simulink model "Plant_Model_Gathering"  (R2023a)
settings: Solver=VariableStepAuto  StartTime=0.0  StopTime=10.0  RelTol=1e-3
undefined symbols (not defined in the file): Amps, Ax, Ay, b, d, g, Ion, Ixx, Izz, Jr, Lithium, m, PD
libraries: simulink x5, spsBatteryLib x1, spsControlledCurrentSourceLib x1, spsCurrentMeasurementLib x1
settings Model: Creator=NADJICH  LastModifiedBy=NADJICH

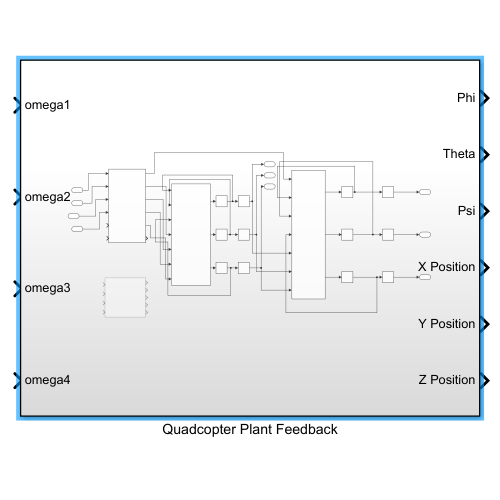
[thumbnail: Simulink's stored preview of the top-level diagram]
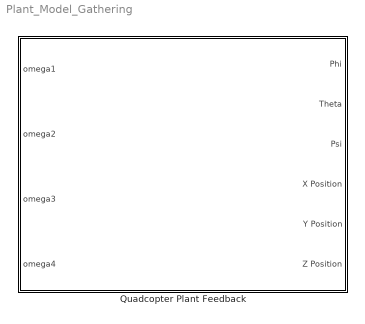
== system Plant_Model_Gathering ==
  Quadcopter Plant Feedback : Subsystem

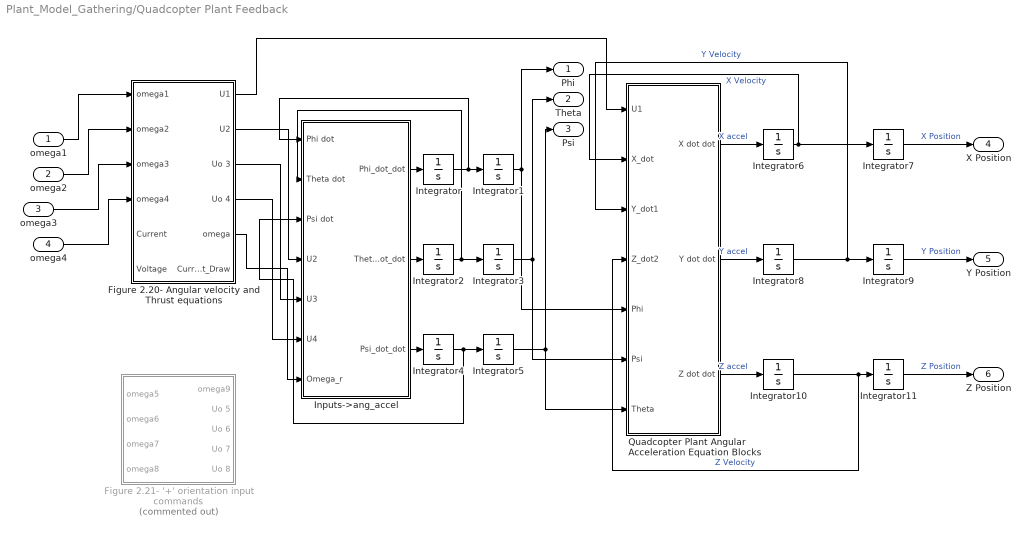
== system Plant_Model_Gathering/Quadcopter Plant Feedback ==
  omega1 : Inport
  omega2 : Inport  Port=2
  omega3 : Inport  Port=3
  omega4 : Inport  Port=4
  Figure 2.20- Angular velocity and Thrust equations : Subsystem
  Figure 2.21- '+' orientation input commands : Subsystem  Commented=on
  Inputs->ang_accel : Subsystem
  Integrator{,2,4,6..10} (8 alike) : Integrator
  Integrator1 : Integrator  WrapState=on
  Integrator11 : Integrator  LimitOutput=on  UpperSaturationLimit=0
  Integrator3 : Integrator  WrapState=on
  Integrator5 : Integrator  WrapState=on
  Quadcopter Plant Angular Acceleration Equation Blocks : Subsystem
  Phi : Outport
  Theta : Outport  Port=2
  Psi : Outport  Port=3
  X Position : Outport  Port=4
  Y Position : Outport  Port=5
  Z Position : Outport  Port=6
  wires:
  omega1/1 -> Figure 2.20- Angular velocity and Thrust equations/1(omega1)
  omega2/1 -> Figure 2.20- Angular velocity and Thrust equations/2(omega2)
  omega3/1 -> Figure 2.20- Angular velocity and Thrust equations/3(omega3)
  omega4/1 -> Figure 2.20- Angular velocity and Thrust equations/4(omega4)
  Figure 2.20- Angular velocity and Thrust equations/5(omega) -> Inputs->ang_accel/7(Omega_r)
  Figure 2.20- Angular velocity and Thrust equations/2(U2) -> Inputs->ang_accel/4(U2)
  Figure 2.20- Angular velocity and Thrust equations/3(Uo 3) -> Inputs->ang_accel/5(U3)
  Figure 2.20- Angular velocity and Thrust equations/4(Uo 4) -> Inputs->ang_accel/6(U4)
  Inputs->ang_accel/1(Phi_dot_dot) -> Integrator/1
  Integrator/1 -> Integrator1/1, Inputs->ang_accel/1(Phi dot)
  Integrator2/1 -> Integrator3/1, Inputs->ang_accel/2(Theta dot)
  Integrator4/1 -> Integrator5/1, Inputs->ang_accel/3(Psi dot)
  Inputs->ang_accel/2(Theta_dot_dot) -> Integrator2/1
  Inputs->ang_accel/3(Psi_dot_dot) -> Integrator4/1
  Integrator1/1 -> Phi/1, Quadcopter Plant Angular Acceleration Equation Blocks/5(Phi)
  Integrator3/1 -> Theta/1, Quadcopter Plant Angular Acceleration Equation Blocks/6(Psi)
  Integrator5/1 -> Psi/1, Quadcopter Plant Angular Acceleration Equation Blocks/7(Theta)
  Figure 2.20- Angular velocity and Thrust equations/1(U1) -> Quadcopter Plant Angular Acceleration Equation Blocks/1(U1)
  Quadcopter Plant Angular Acceleration Equation Blocks/1(X dot dot) -> Integrator6/1  "X accel"
  Quadcopter Plant Angular Acceleration Equation Blocks/2(Y dot dot) -> Integrator8/1  "Y accel"
  Quadcopter Plant Angular Acceleration Equation Blocks/3(Z dot dot) -> Integrator10/1  "Z accel"
  Integrator6/1 -> Quadcopter Plant Angular Acceleration Equation Blocks/2(X_dot), Integrator7/1  "X Velocity"
  Integrator7/1 -> X Position/1  "X Position"
  Integrator8/1 -> Quadcopter Plant Angular Acceleration Equation Blocks/3(Y_dot1), Integrator9/1  "Y Velocity"
  Integrator9/1 -> Y Position/1  "Y Position"
  Integrator10/1 -> Integrator11/1, Quadcopter Plant Angular Acceleration Equation Blocks/4(Z_dot2)  "Z Velocity"
  Integrator11/1 -> Z Position/1  "Z Position"

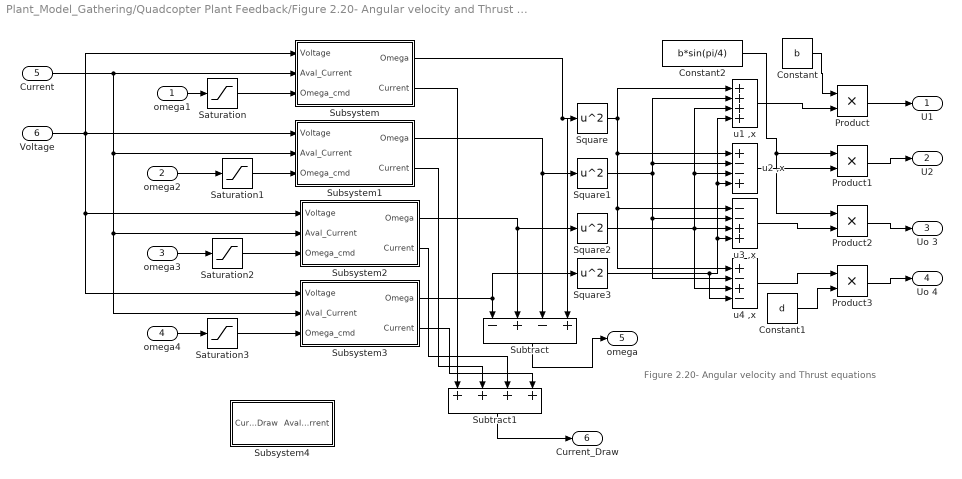
== system Plant_Model_Gathering/Quadcopter Plant Feedback/Figure 2.20- Angular velocity and Thrust equations ==
  note: Figure 2.20- Angular velocity and Thrust equations
  omega1 : Inport
  omega2 : Inport  Port=2
  omega3 : Inport  Port=3
  omega4 : Inport  Port=4
  Current : Inport  Port=5
  Voltage : Inport  Port=6
  Constant : Constant  Value=b
  Constant1 : Constant  Value=d
  Constant2 : Constant  Value=b*sin(pi/4)
  Product{,1..3} (4 alike) : Product
  Saturation{,1..3} (4 alike) : Saturate  UpperLimit=inf  LowerLimit=0
  Square{,1..3} (4 alike) : Math  Operator=square
  Subsystem : Subsystem  mask{Jr=6.5e-7, b_m=2.415-6, Kemf=0.00255, Kt=0.00255, R=0.117, L=1.17e-4}
  Subsystem1 : Subsystem  mask{Jr=6.5e-7, b_m=2.415-6, Kemf=0.00255, Kt=0.00255, R=0.117, L=1.17e-4}
  Subsystem2 : Subsystem  mask{Jr=6.5e-7, b_m=2.415-6, Kemf=0.00255, Kt=0.00255, R=0.117, L=1.17e-4}
  Subsystem3 : Subsystem  mask{Jr=6.5e-7, b_m=2.415-6, Kemf=0.00255, Kt=0.00255, R=0.117, L=1.17e-4}
  Subsystem4 : Subsystem
  Subtract : Sum  Inputs=-+-+
  Subtract1 : Sum  Inputs=++++
  u1 ,x : Sum  Inputs=++++
  u2 ,x : Sum  Inputs=+--+
  u3 ,x : Sum  Inputs=--++
  u4 ,x : Sum  Inputs=+-+-
  U1 : Outport
  U2 : Outport  Port=2
  Uo 3 : Outport  Port=3
  Uo 4 : Outport  Port=4
  omega : Outport  Port=5
  Current_Draw : Outport  Port=6
  wires:
  Constant/1 -> Product/1
  Product1/1 -> U2/1
  u4 ,x/1 -> Product3/1
  Square3/1 -> u4 ,x/4, u3 ,x/4, u2 ,x/4, u1 ,x/4
  omega1/1 -> Saturation/1
  Product/1 -> U1/1
  Square1/1 -> u2 ,x/2, u1 ,x/2, u4 ,x/2, u3 ,x/2
  u3 ,x/1 -> Product2/2
  u1 ,x/1 -> Product/2
  Constant1/1 -> Product3/2
  Constant2/1 -> Product1/1, Product2/1
  Square/1 -> u4 ,x/1, u3 ,x/1, u2 ,x/1, u1 ,x/1
  Square2/1 -> u4 ,x/3, u3 ,x/3, u1 ,x/3, u2 ,x/3
  Product2/1 -> Uo 3/1
  Subtract/1 -> omega/1
  Product3/1 -> Uo 4/1
  u2 ,x/1 -> Product1/2
  omega2/1 -> Saturation1/1
  omega3/1 -> Saturation2/1
  omega4/1 -> Saturation3/1
  Subsystem/1(Omega) -> Square/1, Subtract/4
  Subsystem1/1(Omega) -> Subtract/3, Square1/1
  Subsystem2/1(Omega) -> Subtract/2, Square2/1
  Subsystem3/1(Omega) -> Square3/1, Subtract/1
  Subsystem/2(Current) -> Subtract1/1
  Subsystem1/2(Current) -> Subtract1/2
  Subsystem2/2(Current) -> Subtract1/3
  Subsystem3/2(Current) -> Subtract1/4
  Subtract1/1 -> Current_Draw/1
  Current/1 -> Subsystem/2(Aval_Current), Subsystem1/2(Aval_Current), Subsystem2/2(Aval_Current), Subsystem3/2(Aval_Current)
  Voltage/1 -> Subsystem/1(Voltage), Subsystem1/1(Voltage), Subsystem2/1(Voltage), Subsystem3/1(Voltage)
  Saturation/1 -> Subsystem/3(Omega_cmd)
  Saturation1/1 -> Subsystem1/3(Omega_cmd)
  Saturation2/1 -> Subsystem2/3(Omega_cmd)
  Saturation3/1 -> Subsystem3/3(Omega_cmd)

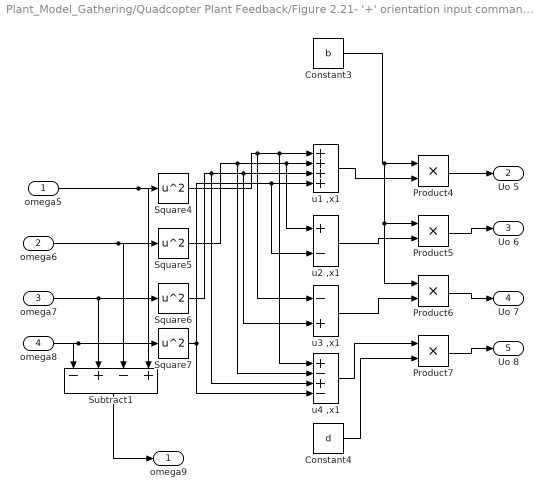
== system Plant_Model_Gathering/Quadcopter Plant Feedback/Figure 2.21- '+' orientation input commands ==
  omega5 : Inport
  omega6 : Inport  Port=2
  omega7 : Inport  Port=3
  omega8 : Inport  Port=4
  Constant3 : Constant  Value=b
  Constant4 : Constant  Value=d
  Product{4..7} (4 alike) : Product
  Square{4..7} (4 alike) : Math  Operator=square
  Subtract1 : Sum  Inputs=-+-+
  u1 ,x1 : Sum  Inputs=++++
  u2 ,x1 : Sum  Inputs=+-
  u3 ,x1 : Sum  Inputs=-+
  u4 ,x1 : Sum  Inputs=+-+-
  omega9 : Outport
  Uo 5 : Outport  Port=2
  Uo 6 : Outport  Port=3
  Uo 7 : Outport  Port=4
  Uo 8 : Outport  Port=5
  wires:
  Square5/1 -> u4 ,x1/2, u2 ,x1/1, u1 ,x1/2
  Constant3/1 -> Product6/1, Product5/1, Product4/1
  Square4/1 -> u3 ,x1/1, u4 ,x1/1, u1 ,x1/1
  Product7/1 -> Uo 8/1
  Constant4/1 -> Product7/2
  omega6/1 -> Square5/1, Subtract1/3
  Product5/1 -> Uo 6/1
  Square7/1 -> u2 ,x1/2, u1 ,x1/4, u4 ,x1/4
  Product4/1 -> Uo 5/1
  u1 ,x1/1 -> Product4/2
  Square6/1 -> u4 ,x1/3, u3 ,x1/2, u1 ,x1/3
  omega8/1 -> Square7/1, Subtract1/1
  u2 ,x1/1 -> Product5/2
  Subtract1/1 -> omega9/1
  omega7/1 -> Square6/1, Subtract1/2
  omega5/1 -> Subtract1/4, Square4/1
  u3 ,x1/1 -> Product6/2
  Product6/1 -> Uo 7/1
  u4 ,x1/1 -> Product7/1

== system Plant_Model_Gathering/Quadcopter Plant Feedback/Inputs->ang_accel ==
  Phi dot : Inport
  Theta dot : Inport  Port=2
  Psi dot : Inport  Port=3
  U2 : Inport  Port=4
  U3 : Inport  Port=5
  U4 : Inport  Port=6
  Omega_r : Inport  Port=7
  Subsystem2 : Subsystem
  Subsystem3 : Subsystem
  Subsystem4 : Subsystem
  Phi_dot_dot : Outport
  Theta_dot_dot : Outport  Port=2
  Psi_dot_dot : Outport  Port=3
  wires:
  Subsystem4/1(Psi_dot_dot) -> Psi_dot_dot/1
  Psi dot/1 -> Subsystem3/4(Omega_r), Subsystem2/4(Psi dot)
  Phi dot/1 -> Subsystem3/2(Phi dot), Subsystem4/3(Phi dot)
  Omega_r/1 -> Subsystem3/1(Psi dot), Subsystem2/2(omega)
  Subsystem3/1(Theta_dot_dot) -> Theta_dot_dot/1
  Subsystem2/1(Phi_dot_dot) -> Phi_dot_dot/1
  Theta dot/1 -> Subsystem2/3(Theta dot), Subsystem4/2(Theta dot)
  U4/1 -> Subsystem4/1(In1)
  U2/1 -> Subsystem2/1(U2)
  U3/1 -> Subsystem3/3(U3)

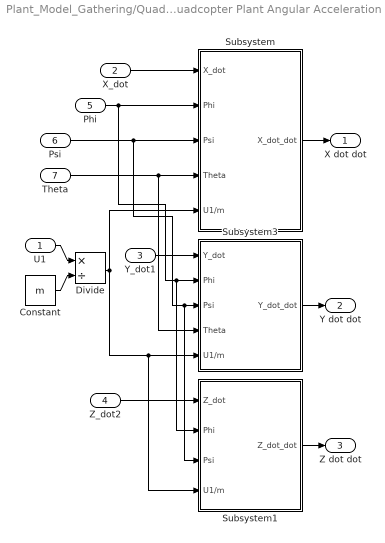
== system Plant_Model_Gathering/Quadcopter Plant Feedback/Quadcopter Plant Angular Acceleration Equation Blocks ==
  U1 : Inport
  X_dot : Inport  Port=2
  Y_dot1 : Inport  Port=3
  Z_dot2 : Inport  Port=4
  Phi : Inport  Port=5
  Psi : Inport  Port=6
  Theta : Inport  Port=7
  Constant : Constant  Value=m
  Divide : Product  Inputs=*/
  Subsystem : Subsystem
  Subsystem1 : Subsystem
  Subsystem3 : Subsystem
  X dot dot : Outport
  Y dot dot : Outport  Port=2
  Z dot dot : Outport  Port=3
  wires:
  Subsystem3/1(Y_dot_dot) -> Y dot dot/1
  U1/1 -> Divide/1
  Constant/1 -> Divide/2
  Subsystem/1(X_dot_dot) -> X dot dot/1
  Subsystem1/1(Z_dot_dot) -> Z dot dot/1
  X_dot/1 -> Subsystem/1(X_dot)
  Divide/1 -> Subsystem1/4(U1/m), Subsystem3/5(U1/m), Subsystem/5(U1/m)
  Y_dot1/1 -> Subsystem3/1(Y_dot)
  Phi/1 -> Subsystem1/2(Phi), Subsystem3/2(Phi), Subsystem/2(Phi)
  Theta/1 -> Subsystem3/4(Theta), Subsystem/4(Theta)
  Psi/1 -> Subsystem1/3(Psi), Subsystem3/3(Psi), Subsystem/3(Psi)
  Z_dot2/1 -> Subsystem1/1(Z_dot)

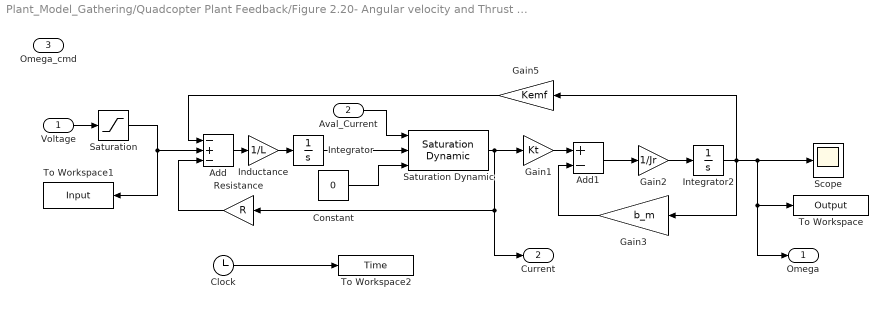
== system Plant_Model_Gathering/Quadcopter Plant Feedback/Figure 2.20- Angular velocity and Thrust equations/Subsystem ==
  Voltage : Inport
  Aval_Current : Inport  Port=2
  Omega_cmd : Inport  Port=3
  Add : Sum  Inputs=-+-
  Add1 : Sum  Inputs=+-
  Clock : Clock
  Constant : Constant  Value=0
  Gain1 : Gain  Gain=Kt
  Gain2 : Gain  Gain=1/Jr
  Gain3 : Gain  Gain=b_m
  Gain5 : Gain  Gain=Kemf
  Inductance : Gain  Gain=1/L
  Integrator : Integrator  LimitOutput=on  UpperSaturationLimit=0
  Integrator2 : Integrator  LimitOutput=on  UpperSaturationLimit=0
  Resistance : Gain  Gain=R
  Saturation : Saturate
  Saturation Dynamic : simulink/Discontinuities/Saturation Dynamic  OutMin=[]  OutMax=[]  OutDataTypeStr=Inherit: Same as second input  OutDataType=fixdt(1, 16)  OutScaling=2^-10  DoSatur=off
  Scope : Scope
  To Workspace : ToWorkspace  VariableName=Output  SampleTime=-1
  To Workspace1 : ToWorkspace  VariableName=Input  SampleTime=-1
  To Workspace2 : ToWorkspace  VariableName=Time  SampleTime=-1
  Omega : Outport
  Current : Outport  Port=2
  wires:
  Voltage/1 -> Saturation/1
  Integrator/1 -> Saturation Dynamic/2
  Integrator2/1 -> Scope/1, Omega/1, To Workspace/1, Gain3/1, Gain5/1
  Add/1 -> Inductance/1
  Gain2/1 -> Integrator2/1
  Gain5/1 -> Add/1
  Gain3/1 -> Add1/2
  Add1/1 -> Gain2/1
  Resistance/1 -> Add/3
  Inductance/1 -> Integrator/1
  Gain1/1 -> Add1/1
  Saturation/1 -> Add/2, To Workspace1/1
  Clock/1 -> To Workspace2/1
  Saturation Dynamic/1 -> Current/1, Resistance/1, Gain1/1
  Constant/1 -> Saturation Dynamic/3
  Aval_Current/1 -> Saturation Dynamic/1

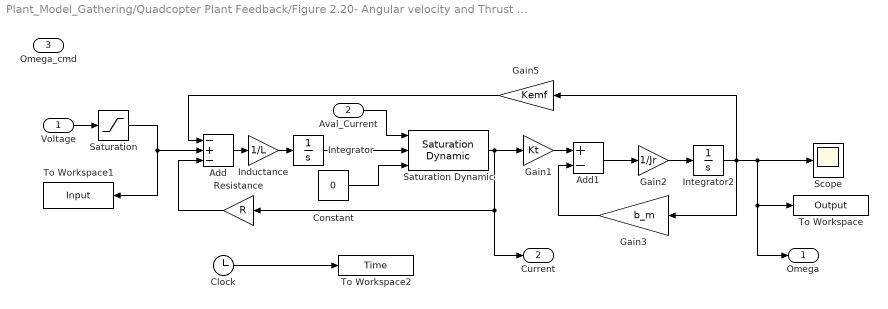
== system Plant_Model_Gathering/Quadcopter Plant Feedback/Figure 2.20- Angular velocity and Thrust equations/Subsystem1 ==
  Voltage : Inport
  Aval_Current : Inport  Port=2
  Omega_cmd : Inport  Port=3
  Add : Sum  Inputs=-+-
  Add1 : Sum  Inputs=+-
  Clock : Clock
  Constant : Constant  Value=0
  Gain1 : Gain  Gain=Kt
  Gain2 : Gain  Gain=1/Jr
  Gain3 : Gain  Gain=b_m
  Gain5 : Gain  Gain=Kemf
  Inductance : Gain  Gain=1/L
  Integrator : Integrator  LimitOutput=on  UpperSaturationLimit=0
  Integrator2 : Integrator  LimitOutput=on  UpperSaturationLimit=0
  Resistance : Gain  Gain=R
  Saturation : Saturate
  Saturation Dynamic : simulink/Discontinuities/Saturation Dynamic  OutMin=[]  OutMax=[]  OutDataTypeStr=Inherit: Same as second input  OutDataType=fixdt(1, 16)  OutScaling=2^-10  DoSatur=off
  Scope : Scope
  To Workspace : ToWorkspace  VariableName=Output  SampleTime=-1
  To Workspace1 : ToWorkspace  VariableName=Input  SampleTime=-1
  To Workspace2 : ToWorkspace  VariableName=Time  SampleTime=-1
  Omega : Outport
  Current : Outport  Port=2
  wires:
  Aval_Current/1 -> Saturation Dynamic/1
  Constant/1 -> Saturation Dynamic/3
  Saturation Dynamic/1 -> Gain1/1, Resistance/1, Current/1
  Clock/1 -> To Workspace2/1
  Saturation/1 -> To Workspace1/1, Add/2
  Gain1/1 -> Add1/1
  Inductance/1 -> Integrator/1
  Resistance/1 -> Add/3
  Add1/1 -> Gain2/1
  Gain3/1 -> Add1/2
  Gain5/1 -> Add/1
  Gain2/1 -> Integrator2/1
  Add/1 -> Inductance/1
  Integrator2/1 -> Gain5/1, Gain3/1, To Workspace/1, Omega/1, Scope/1
  Integrator/1 -> Saturation Dynamic/2
  Voltage/1 -> Saturation/1

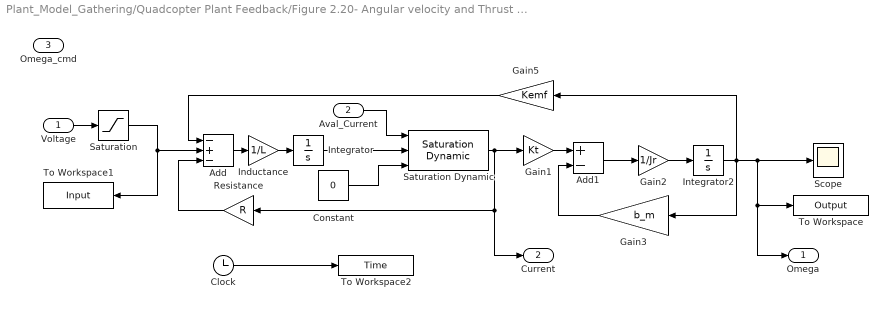
== system Plant_Model_Gathering/Quadcopter Plant Feedback/Figure 2.20- Angular velocity and Thrust equations/Subsystem2 ==
  Voltage : Inport
  Aval_Current : Inport  Port=2
  Omega_cmd : Inport  Port=3
  Add : Sum  Inputs=-+-
  Add1 : Sum  Inputs=+-
  Clock : Clock
  Constant : Constant  Value=0
  Gain1 : Gain  Gain=Kt
  Gain2 : Gain  Gain=1/Jr
  Gain3 : Gain  Gain=b_m
  Gain5 : Gain  Gain=Kemf
  Inductance : Gain  Gain=1/L
  Integrator : Integrator  LimitOutput=on  UpperSaturationLimit=0
  Integrator2 : Integrator  LimitOutput=on  UpperSaturationLimit=0
  Resistance : Gain  Gain=R
  Saturation : Saturate
  Saturation Dynamic : simulink/Discontinuities/Saturation Dynamic  OutMin=[]  OutMax=[]  OutDataTypeStr=Inherit: Same as second input  OutDataType=fixdt(1, 16)  OutScaling=2^-10  DoSatur=off
  Scope : Scope
  To Workspace : ToWorkspace  VariableName=Output  SampleTime=-1
  To Workspace1 : ToWorkspace  VariableName=Input  SampleTime=-1
  To Workspace2 : ToWorkspace  VariableName=Time  SampleTime=-1
  Omega : Outport
  Current : Outport  Port=2
  wires:
  Voltage/1 -> Saturation/1
  Integrator/1 -> Saturation Dynamic/2
  Integrator2/1 -> Scope/1, Omega/1, To Workspace/1, Gain3/1, Gain5/1
  Add/1 -> Inductance/1
  Gain2/1 -> Integrator2/1
  Gain5/1 -> Add/1
  Gain3/1 -> Add1/2
  Add1/1 -> Gain2/1
  Resistance/1 -> Add/3
  Inductance/1 -> Integrator/1
  Gain1/1 -> Add1/1
  Saturation/1 -> Add/2, To Workspace1/1
  Clock/1 -> To Workspace2/1
  Saturation Dynamic/1 -> Current/1, Resistance/1, Gain1/1
  Constant/1 -> Saturation Dynamic/3
  Aval_Current/1 -> Saturation Dynamic/1

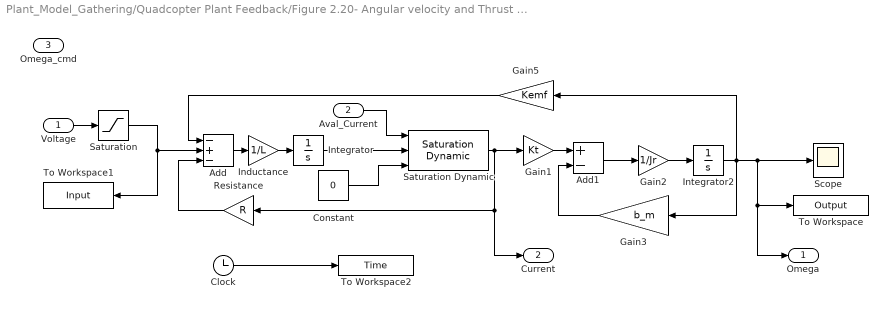
== system Plant_Model_Gathering/Quadcopter Plant Feedback/Figure 2.20- Angular velocity and Thrust equations/Subsystem3 ==
  Voltage : Inport
  Aval_Current : Inport  Port=2
  Omega_cmd : Inport  Port=3
  Add : Sum  Inputs=-+-
  Add1 : Sum  Inputs=+-
  Clock : Clock
  Constant : Constant  Value=0
  Gain1 : Gain  Gain=Kt
  Gain2 : Gain  Gain=1/Jr
  Gain3 : Gain  Gain=b_m
  Gain5 : Gain  Gain=Kemf
  Inductance : Gain  Gain=1/L
  Integrator : Integrator  LimitOutput=on  UpperSaturationLimit=0
  Integrator2 : Integrator  LimitOutput=on  UpperSaturationLimit=0
  Resistance : Gain  Gain=R
  Saturation : Saturate
  Saturation Dynamic : simulink/Discontinuities/Saturation Dynamic  OutMin=[]  OutMax=[]  OutDataTypeStr=Inherit: Same as second input  OutDataType=fixdt(1, 16)  OutScaling=2^-10  DoSatur=off
  Scope : Scope
  To Workspace : ToWorkspace  VariableName=Output  SampleTime=-1
  To Workspace1 : ToWorkspace  VariableName=Input  SampleTime=-1
  To Workspace2 : ToWorkspace  VariableName=Time  SampleTime=-1
  Omega : Outport
  Current : Outport  Port=2
  wires:
  Aval_Current/1 -> Saturation Dynamic/1
  Constant/1 -> Saturation Dynamic/3
  Saturation Dynamic/1 -> Gain1/1, Resistance/1, Current/1
  Clock/1 -> To Workspace2/1
  Saturation/1 -> To Workspace1/1, Add/2
  Gain1/1 -> Add1/1
  Inductance/1 -> Integrator/1
  Resistance/1 -> Add/3
  Add1/1 -> Gain2/1
  Gain3/1 -> Add1/2
  Gain5/1 -> Add/1
  Gain2/1 -> Integrator2/1
  Add/1 -> Inductance/1
  Integrator2/1 -> Gain5/1, Gain3/1, To Workspace/1, Omega/1, Scope/1
  Integrator/1 -> Saturation Dynamic/2
  Voltage/1 -> Saturation/1

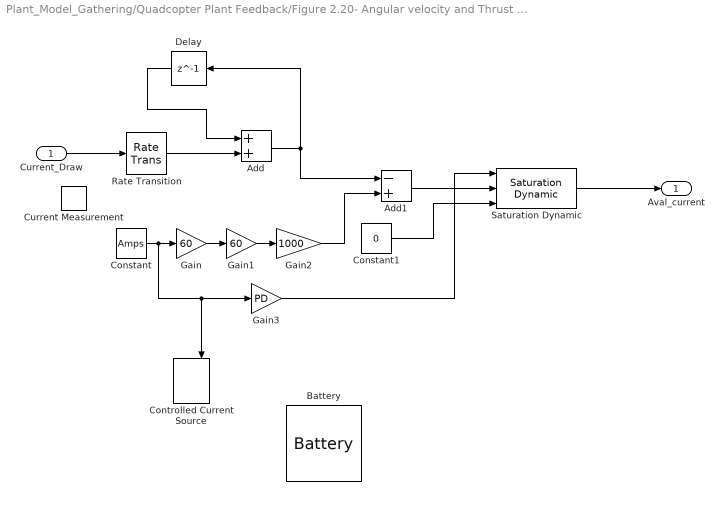
== system Plant_Model_Gathering/Quadcopter Plant Feedback/Figure 2.20- Angular velocity and Thrust equations/Subsystem4 ==
  Current_Draw : Inport
  Add : Sum
  Add1 : Sum  Inputs=-+
  Battery : spsBatteryLib/Battery  BatType=Lithium-Ion  ShowTempParam=off  ThermalPreset=no  ShowAgeParam=off  NomV=10  NomQ=0.7  SOC=100  Batt_Tr=30  PresetModel=on  MaxQ=0.7  MinV=7.5  FullV=11.6399  Dis_rate=0.30435  R=0.14286  Normal_OP=0.63304  expZone="[10.8039    0.0343913]"  current=[6.5 13 32.5]  Units=Time  Tci=20  NomT=20  T2=-30  MaxQ2=4.8  FullV2=7.1  Normal_OP2=5.655  expZone2="[6.58           1]"  Rca=0.6  ti=2000  Dp=0  Neq0=0  Tsim=1e6  Ta1=25  Qeol=5.4*0.9  Reol=0.013333*1.2  Char_age=[2.3478, 3]  Dis_age=[2.3478, 10]  N1=1500  N2=10500  N3=1000  N4=1400  Ta2=45  N5=950
  Constant : Constant  Value=Amps
  Constant1 : Constant  Value=0
  Controlled Current Source : spsControlledCurrentSourceLib/Controlled Current Source  Initialize=on  Source_Type=AC  Amplitude=0  Phase=0  Frequency=0  Measurements=None
  Current Measurement : spsCurrentMeasurementLib/Current Measurement  PhasorSimulation=off  OutputType=Complex  PSBequivalent=0
  Delay : Delay  DelayLength=1
  Gain : Gain  Gain=60
  Gain1 : Gain  Gain=60
  Gain2 : Gain  Gain=1000
  Gain3 : Gain  Gain=PD
  Rate Transition : RateTransition
  Saturation Dynamic : simulink/Discontinuities/Saturation Dynamic  OutMin=[]  OutMax=[]  OutDataTypeStr=Inherit: Same as second input  OutDataType=fixdt(1, 16)  OutScaling=2^-10  DoSatur=off
  Aval_current : Outport
  wires:
  Current_Draw/1 -> Rate Transition/1
  Add/1 -> Delay/1, Add1/1
  Delay/1 -> Add/1
  Rate Transition/1 -> Add/2
  Gain/1 -> Gain1/1
  Gain1/1 -> Gain2/1
  Constant/1 -> Controlled Current Source/1, Gain3/1, Gain/1
  Gain2/1 -> Add1/2
  Add1/1 -> Saturation Dynamic/2
  Gain3/1 -> Saturation Dynamic/1
  Constant1/1 -> Saturation Dynamic/3
  Saturation Dynamic/1 -> Aval_current/1

== system Plant_Model_Gathering/Quadcopter Plant Feedback/Inputs->ang_accel/Subsystem2 ==
  U2 : Inport
  omega : Inport  Port=2
  Theta dot : Inport  Port=3
  Psi dot : Inport  Port=4
  Add : Sum  Inputs=+++
  Constant : Constant
  Constant1 : Constant  Value=Jr
  Constant2 : Constant  Value=Izz-Ixx
  Constant3 : Constant
  Divide : Product  Inputs=*/
  Product : Product
  Product1 : Product  Inputs=3
  Product2 : Product  Inputs=3
  Phi_dot_dot : Outport
  wires:
  Add/1 -> Divide/1
  Divide/1 -> Phi_dot_dot/1
  Constant2/1 -> Product2/3
  Product2/1 -> Add/3
  U2/1 -> Product/2
  Product/1 -> Add/1
  Constant/1 -> Product/1
  Product1/1 -> Add/2
  Constant1/1 -> Product1/1
  Constant3/1 -> Divide/2
  omega/1 -> Product1/2
  Theta dot/1 -> Product2/1, Product1/3
  Psi dot/1 -> Product2/2

== system Plant_Model_Gathering/Quadcopter Plant Feedback/Inputs->ang_accel/Subsystem3 ==
  Psi dot : Inport
  Phi dot : Inport  Port=2
  U3 : Inport  Port=3
  Omega_r : Inport  Port=4
  Add2 : Sum  Inputs=+++
  Constant11 : Constant
  Constant12 : Constant  Value=Izz-Ixx
  Constant8 : Constant
  Constant9 : Constant  Value=Jr
  Divide2 : Product  Inputs=*/
  Product6 : Product
  Product7 : Product  Inputs=3
  Product8 : Product  Inputs=3
  Theta_dot_dot : Outport
  wires:
  Divide2/1 -> Theta_dot_dot/1
  Product7/1 -> Add2/2
  Add2/1 -> Divide2/1
  Constant9/1 -> Product7/1
  Product8/1 -> Add2/3
  Constant12/1 -> Product8/3
  Constant11/1 -> Divide2/2
  Product6/1 -> Add2/1
  Constant8/1 -> Product6/1
  Phi dot/1 -> Product7/3, Product8/1
  Psi dot/1 -> Product8/2
  Omega_r/1 -> Product7/2
  U3/1 -> Product6/2

== system Plant_Model_Gathering/Quadcopter Plant Feedback/Inputs->ang_accel/Subsystem4 ==
  In1 : Inport
  Theta dot : Inport  Port=2
  Phi dot : Inport  Port=3
  Add1 : Sum
  Constant10 : Constant  Value=Izz-Ixx
  Constant7 : Constant
  Divide1 : Product  Inputs=*/
  Product4 : Product  Inputs=3
  Psi_dot_dot : Outport
  wires:
  Constant10/1 -> Product4/3
  Product4/1 -> Add1/2
  Divide1/1 -> Psi_dot_dot/1
  In1/1 -> Add1/1
  Constant7/1 -> Divide1/2
  Add1/1 -> Divide1/1
  Phi dot/1 -> Product4/2
  Theta dot/1 -> Product4/1

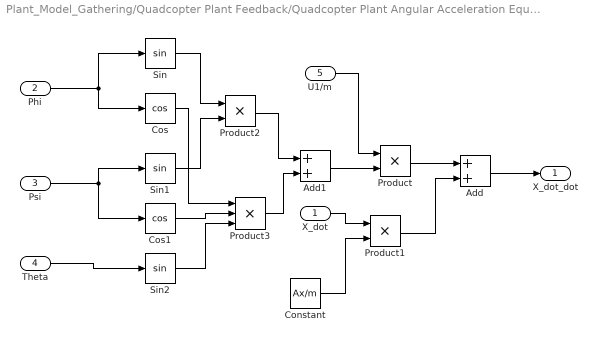
== system Plant_Model_Gathering/Quadcopter Plant Feedback/Quadcopter Plant Angular Acceleration Equation Blocks/Subsystem ==
  X_dot : Inport
  Phi : Inport  Port=2
  Psi : Inport  Port=3
  Theta : Inport  Port=4
  U1/m : Inport  Port=5
  Add : Sum
  Add1 : Sum
  Constant : Constant  Value=Ax/m
  Cos : Trigonometry  Operator=cos
  Cos1 : Trigonometry  Operator=cos
  Product : Product
  Product1 : Product
  Product2 : Product
  Product3 : Product  Inputs=3
  Sin : Trigonometry
  Sin1 : Trigonometry
  Sin2 : Trigonometry
  X_dot_dot : Outport
  wires:
  Phi/1 -> Sin/1, Cos/1
  Psi/1 -> Cos1/1, Sin1/1
  Theta/1 -> Sin2/1
  Sin1/1 -> Product2/2
  Sin/1 -> Product2/1
  Cos/1 -> Product3/1
  Cos1/1 -> Product3/2
  Sin2/1 -> Product3/3
  Product3/1 -> Add1/2
  Product2/1 -> Add1/1
  Add1/1 -> Product/2
  U1/m/1 -> Product/1
  X_dot/1 -> Product1/1
  Constant/1 -> Product1/2
  Product1/1 -> Add/2
  Product/1 -> Add/1
  Add/1 -> X_dot_dot/1

== system Plant_Model_Gathering/Quadcopter Plant Feedback/Quadcopter Plant Angular Acceleration Equation Blocks/Subsystem1 ==
  Z_dot : Inport
  Phi : Inport  Port=2
  Psi : Inport  Port=3
  U1/m : Inport  Port=4
  Add : Sum  Inputs=+-
  Add1 : Sum  Inputs=-+
  Constant : Constant  Value=Ay/m
  Constant1 : Constant  Value=g
  Cos : Trigonometry  Operator=cos
  Cos2 : Trigonometry  Operator=cos
  Product1 : Product
  Product3 : Product  Inputs=3
  Z_dot_dot : Outport
  wires:
  Phi/1 -> Cos/1
  Psi/1 -> Cos2/1
  Cos/1 -> Product3/1
  Product3/1 -> Add1/2
  Z_dot/1 -> Product1/1
  Constant/1 -> Product1/2
  Product1/1 -> Add/2
  Add/1 -> Z_dot_dot/1
  Constant1/1 -> Add1/1
  Cos2/1 -> Product3/2
  U1/m/1 -> Product3/3
  Add1/1 -> Add/1

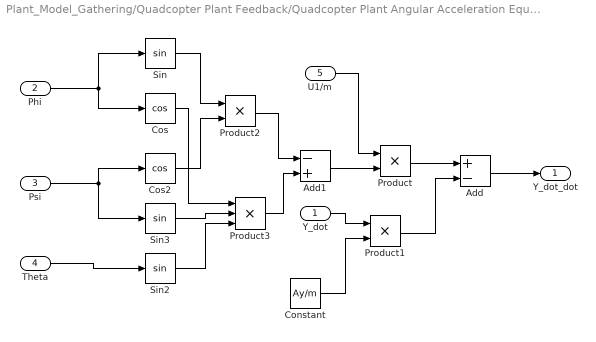
== system Plant_Model_Gathering/Quadcopter Plant Feedback/Quadcopter Plant Angular Acceleration Equation Blocks/Subsystem3 ==
  Y_dot : Inport
  Phi : Inport  Port=2
  Psi : Inport  Port=3
  Theta : Inport  Port=4
  U1/m : Inport  Port=5
  Add : Sum  Inputs=+-
  Add1 : Sum  Inputs=-+
  Constant : Constant  Value=Ay/m
  Cos : Trigonometry  Operator=cos
  Cos2 : Trigonometry  Operator=cos
  Product : Product
  Product1 : Product
  Product2 : Product
  Product3 : Product  Inputs=3
  Sin : Trigonometry
  Sin2 : Trigonometry
  Sin3 : Trigonometry
  Y_dot_dot : Outport
  wires:
  Add/1 -> Y_dot_dot/1
  Product/1 -> Add/1
  Product1/1 -> Add/2
  Constant/1 -> Product1/2
  Y_dot/1 -> Product1/1
  U1/m/1 -> Product/1
  Add1/1 -> Product/2
  Product2/1 -> Add1/1
  Product3/1 -> Add1/2
  Sin2/1 -> Product3/3
  Sin3/1 -> Product3/2
  Cos/1 -> Product3/1
  Sin/1 -> Product2/1
  Cos2/1 -> Product2/2
  Theta/1 -> Sin2/1
  Psi/1 -> Cos2/1, Sin3/1
  Phi/1 -> Cos/1, Sin/1
